simulink model "Griewank"  (R2019a)
settings: Solver=FixedStepAuto  StartTime=0.0  StopTime=size(InputValues_20200610T231852540,1) - 1  FixedStep=1  RelTol=1e-3
model workspace (MAT data in the model file):
  InputValues_20200610T231852540 = [0 0.0245361328125 0.049072265625 0.0736083984375 0.09814453125 0.122680664062 0.147216796875 0.171752929688 0.1962890625 0.220825195312 0.245361328125 0.269897460938 ... (257 elements, 257x1)]
libraries: simulink x1
settings Model: OrderedModelArguments=off  Creator=letras  LastModifiedBy=letras
settings DebuggingCC: IntegerOverflowMsg=none  ParameterOverflowMsg=none  ParameterPrecisionLossMsg=none  IntegerSaturationMsg=none

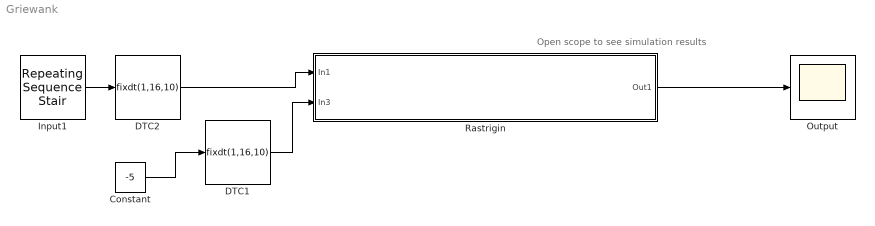
== system Griewank ==
  note: Open scope to see simulation results
  Constant : Constant  Value=-5
  DTC1 : DataTypeConversion  OutDataTypeStr=fixdt(1,16,10)  RndMeth=Nearest
  DTC2 : DataTypeConversion  OutDataTypeStr=fixdt(1,16,10)  RndMeth=Nearest
  Input1 : simulink/Sources/Repeating Sequence Stair  OutValues=[-5 -4.5 -4 -3.5 -3 -2.5 -2 -1.5 -1 -0.5 0 1 2 3 4 5]  tsamp=-1  OutMin=[]  OutMax=[]  OutDataTypeStr=double  OutputDataTypeScalingMode=double  OutDataType=fixdt(0,8)  ConRadixGroup=Best Precision: Vector-wise  OutScaling=2^-12
  Output : Scope
  Rastrigin : Subsystem  Description=This block was created using function approximation.
  wires:
  Rastrigin/1(Out1) -> Output/1
  Input1/1 -> DTC2/1
  DTC2/1 -> Rastrigin/1(In1)
  DTC1/1 -> Rastrigin/2(In3)
  Constant/1 -> DTC1/1

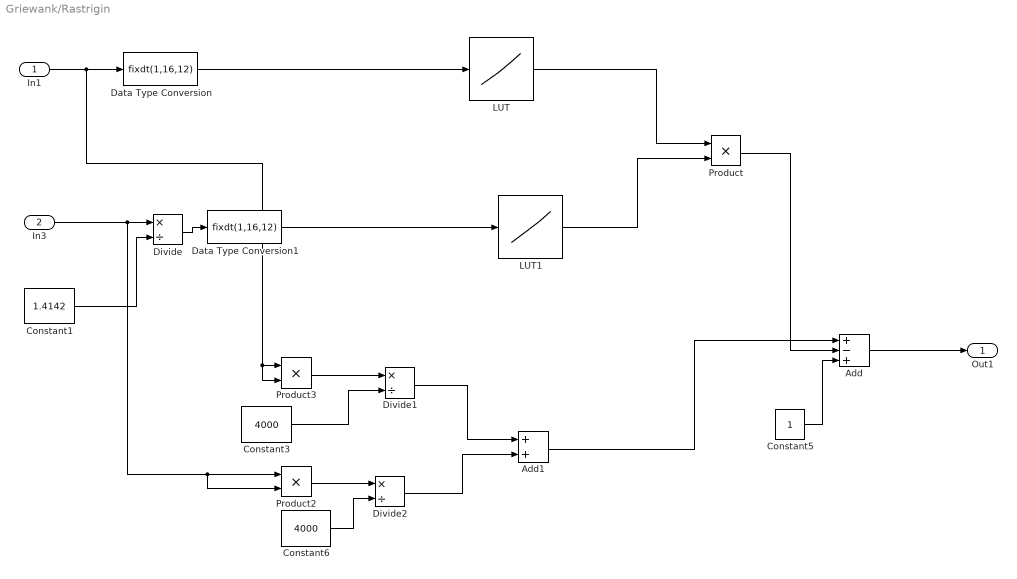
== system Griewank/Rastrigin ==
  In1 : Inport
  In3 : Inport  Port=2
  Add : Sum  Inputs=+-+  OutDataTypeStr=fixdt(1,16,10)
  Add1 : Sum  OutDataTypeStr=fixdt(0,16,10)
  Constant1 : Constant  Value=1.4142  OutDataTypeStr=fixdt(0,16,10)
  Constant3 : Constant  Value=4000  OutDataTypeStr=fixdt(0,16,4)
  Constant5 : Constant  OutDataTypeStr=fixdt(0,16,10)
  Constant6 : Constant  Value=4000  OutDataTypeStr=fixdt(0,16,4)
  Data Type Conversion : DataTypeConversion  OutDataTypeStr=fixdt(1,16,12)
  Data Type Conversion1 : DataTypeConversion  OutDataTypeStr=fixdt(1,16,12)
  Divide : Product  Inputs=*/  RndMeth=Simplest  SaturateOnIntegerOverflow=on
  Divide1 : Product  Inputs=*/  OutDataTypeStr=fixdt(0,16,5)  RndMeth=Simplest  SaturateOnIntegerOverflow=on
  Divide2 : Product  Inputs=*/  OutDataTypeStr=fixdt(0,16,5)  RndMeth=Simplest  SaturateOnIntegerOverflow=on
  LUT : Lookup_n-D  NumberOfTableDimensions=1  LookupTableObject=FunctionApproximation_LUTObject_20210714T214041645  BreakpointsSpecification=Even spacing  BreakpointsForDimension3=[5, 7]  BreakpointsForDimension1FirstPoint=-5  BreakpointsForDimension1DataTypeStr=numerictype(1,16,12)  IndexSearchMethod=Evenly spaced points  Table=[0.28369140625 -0.65362548828125 -0.989990234375 -0.4161376953125 0.540283203125 1 0.540283203125 -0.4161376953125 -0.989990234375 -0.65362548828125 0.28369140625]  TableDataTypeStr=numerictype(1,16,14)  ExtrapMethod=Clip  UseLastTableValue=on  InternalRulePriority=Speed  OutDataTypeStr=numerictype(1,16,14)  RndMeth=Simplest
  LUT1 : Lookup_n-D  NumberOfTableDimensions=1  LookupTableObject=FunctionApproximation_LUTObject_20210714T214041645  BreakpointsSpecification=Even spacing  BreakpointsForDimension3=[5, 7]  BreakpointsForDimension1FirstPoint=-5  BreakpointsForDimension1DataTypeStr=numerictype(1,16,12)  IndexSearchMethod=Evenly spaced points  Table=[0.28369140625 -0.65362548828125 -0.989990234375 -0.4161376953125 0.540283203125 1 0.540283203125 -0.4161376953125 -0.989990234375 -0.65362548828125 0.28369140625]  TableDataTypeStr=numerictype(1,16,14)  ExtrapMethod=Clip  UseLastTableValue=on  InternalRulePriority=Speed  OutDataTypeStr=numerictype(1,16,14)  RndMeth=Simplest
  Product : Product  OutDataTypeStr=fixdt(1,16,13)
  Product2 : Product  OutDataTypeStr=fixdt(0,16,9)
  Product3 : Product  OutDataTypeStr=fixdt(0,16,9)
  Out1 : Outport
  wires:
  Data Type Conversion/1 -> LUT/1
  LUT/1 -> Product/1
  In1/1 -> Product3/2, Product3/1, Data Type Conversion/1
  Data Type Conversion1/1 -> LUT1/1
  In3/1 -> Product2/2, Product2/1, Divide/1
  Constant1/1 -> Divide/2
  Product3/1 -> Divide1/1
  Constant3/1 -> Divide1/2
  Product2/1 -> Divide2/1
  Constant6/1 -> Divide2/2
  Divide1/1 -> Add1/1
  Divide2/1 -> Add1/2
  Add/1 -> Out1/1
  Divide/1 -> Data Type Conversion1/1
  Add1/1 -> Add/1
  Product/1 -> Add/2
  Constant5/1 -> Add/3
  LUT1/1 -> Product/2
